simulink model "SixDofOpenLoop"  (Simulink 8.3)
settings: Solver=ode45  StartTime=0.0  StopTime=10  FixedStep=0.001  RelTol=1e-3
settings Model: Creator=hermanh  LastModifiedBy=USUARIO
settings OptimizationCC: ExpressionDepthLimit=2147483647
settings DebuggingCC: FcnCallInpInsideContextMsg=UseLocalSettings

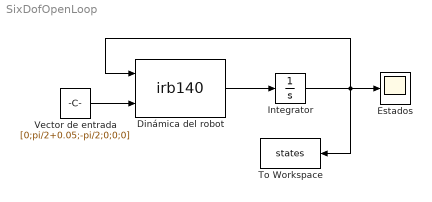
== system SixDofOpenLoop ==
  "\t\tVector de entrada" : Constant  Value=[0;pi/2+0.05;-pi/2;0;0;0]
  Dinámica del robot : M-S-Function  FunctionName=irb140
  Estados : Scope
      settings: SaveName=ScopeData12
  Integrator : Integrator  InitialCondition=[0; 0; pi; 0; pi/2; 0; 0; 0; 0; 0; 0; 0;]
  To Workspace : ToWorkspace  VariableName=states  SaveFormat=Structure With Time  SampleTime=-1
  wires:
  Dinámica del robot/1 -> Integrator/1
  Integrator/1 -> Dinámica del robot/1, Estados/1, To Workspace/1
  "\t\tVector de entrada"/1 -> Dinámica del robot/2
